simulink model "es2_emg_1"  (R2024a)
settings: Solver=VariableStepAuto  StartTime=0.0  StopTime=30  RelTol=1e-3
libraries: vrlib x2
settings Model: Creator=amisq  LastModifiedBy=amisq

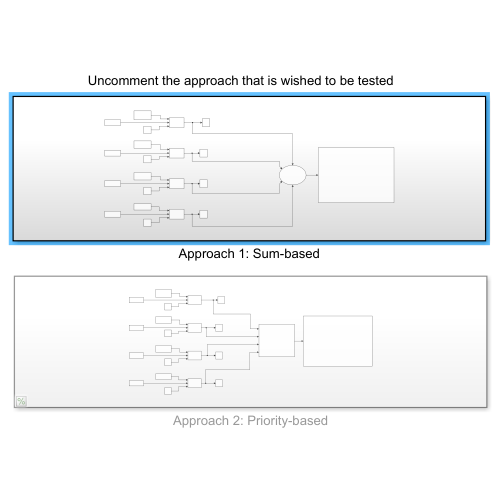
[thumbnail: Simulink's stored preview of the top-level diagram]
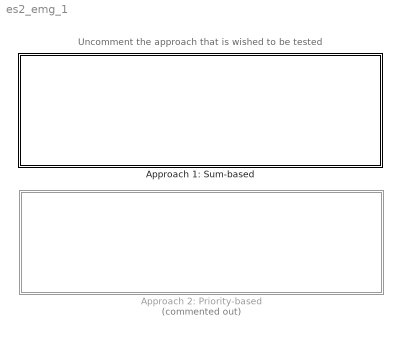
== system es2_emg_1 ==
  note: Uncomment the approach that is wished to be tested
  Approach 1: Sum-based : Subsystem
  Approach 2: Priority-based : Subsystem  Commented=on

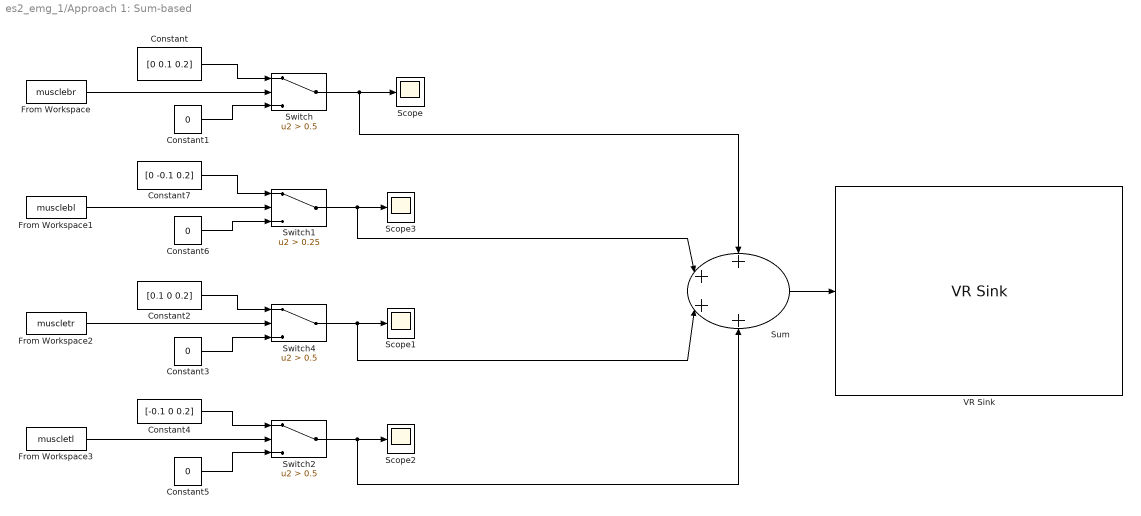
== system es2_emg_1/Approach 1: Sum-based ==
  Constant : Constant  Value=[0 0.1 0.2]
  Constant{1,3,5..6} (4 alike) : Constant  Value=0
  Constant2 : Constant  Value=[0.1 0 0.2]
  Constant4 : Constant  Value=[-0.1 0 0.2]
  Constant7 : Constant  Value=[0 -0.1 0.2]
  From Workspace : FromWorkspace  VariableName=musclebr  SampleTime=0.05
  From Workspace1 : FromWorkspace  VariableName=musclebl  SampleTime=0.05
  From Workspace2 : FromWorkspace  VariableName=muscletr  SampleTime=0.05
  From Workspace3 : FromWorkspace  VariableName=muscletl  SampleTime=0.05
  Scope{,1..3} (4 alike) : Scope
  Sum : Sum  Inputs=++++
  Switch : Switch  Criteria=u2 > Threshold  Threshold=0.5  SaturateOnIntegerOverflow=off  InputSameDT=off
  Switch1 : Switch  Criteria=u2 > Threshold  Threshold=0.25  SaturateOnIntegerOverflow=off  InputSameDT=off
  Switch2 : Switch  Criteria=u2 > Threshold  Threshold=0.5  SaturateOnIntegerOverflow=off  InputSameDT=off
  Switch4 : Switch  Criteria=u2 > Threshold  Threshold=0.5  SaturateOnIntegerOverflow=off  InputSameDT=off
  VR Sink : vrlib/VR Sink  InstantiateOnLoad=on  SampleTime=0.03  ViewEnable=on  RemoteChange=off  RemoteView=off  FieldsWritten=cursor.translation.3.1.1.double  WorldFileName=8_palline_color.wrl  AutoView=off  VideoDimensions=[]  AllowVariableSize=off
  wires:
  Switch2/1 -> Sum/4, Scope2/1
  Constant/1 -> Switch/1
  Switch/1 -> Sum/1, Scope/1
  From Workspace3/1 -> Switch2/2
  Constant2/1 -> Switch4/1
  Switch1/1 -> Sum/2, Scope3/1
  Constant4/1 -> Switch2/1
  Constant6/1 -> Switch1/3
  From Workspace1/1 -> Switch1/2
  Constant5/1 -> Switch2/3
  Constant7/1 -> Switch1/1
  Constant3/1 -> Switch4/3
  From Workspace2/1 -> Switch4/2
  Switch4/1 -> Sum/3, Scope1/1
  From Workspace/1 -> Switch/2
  Sum/1 -> VR Sink/1
  Constant1/1 -> Switch/3

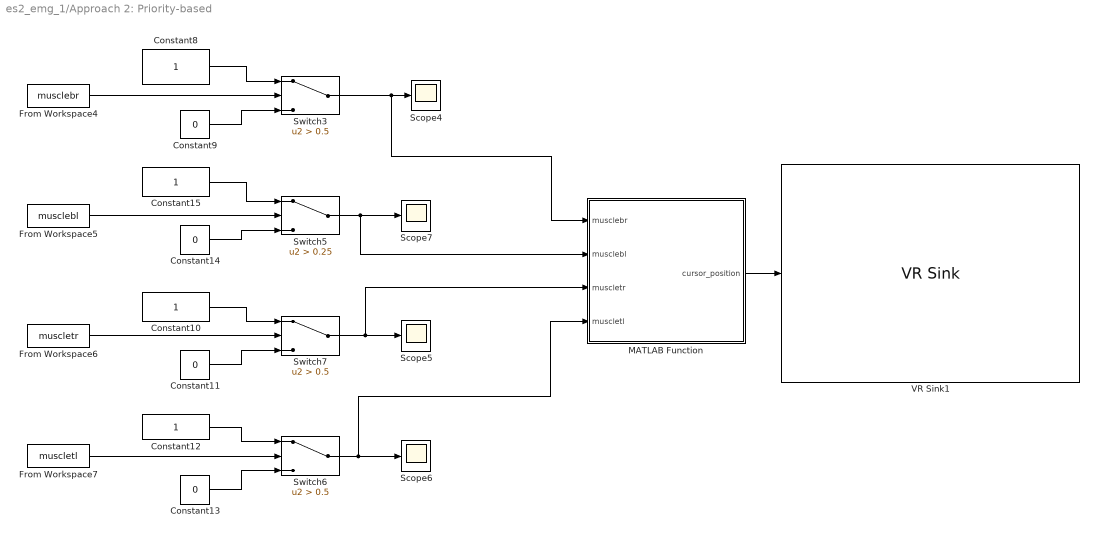
== system es2_emg_1/Approach 2: Priority-based ==
  Constant{8,10,12,15} (4 alike) : Constant
  Constant{9,11,13..14} (4 alike) : Constant  Value=0
  From Workspace4 : FromWorkspace  VariableName=musclebr  SampleTime=0.05
  From Workspace5 : FromWorkspace  VariableName=musclebl  SampleTime=0.05
  From Workspace6 : FromWorkspace  VariableName=muscletr  SampleTime=0.05
  From Workspace7 : FromWorkspace  VariableName=muscletl  SampleTime=0.05
  MATLAB Function : MATLAB Function  TreatAsAtomicUnit=on
  Scope{4..7} (4 alike) : Scope
  Switch3 : Switch  Criteria=u2 > Threshold  Threshold=0.5  SaturateOnIntegerOverflow=off  InputSameDT=off
  Switch5 : Switch  Criteria=u2 > Threshold  Threshold=0.25  SaturateOnIntegerOverflow=off  InputSameDT=off
  Switch6 : Switch  Criteria=u2 > Threshold  Threshold=0.5  SaturateOnIntegerOverflow=off  InputSameDT=off
  Switch7 : Switch  Criteria=u2 > Threshold  Threshold=0.5  SaturateOnIntegerOverflow=off  InputSameDT=off
  VR Sink1 : vrlib/VR Sink  InstantiateOnLoad=on  SampleTime=0.03  ViewEnable=on  RemoteChange=off  RemoteView=off  FieldsWritten=cursor.translation.3.1.1.double  WorldFileName=8_palline_color.wrl  AutoView=off  VideoDimensions=[]  AllowVariableSize=off
  wires:
  From Workspace4/1 -> Switch3/2
  From Workspace7/1 -> Switch6/2
  Switch6/1 -> MATLAB Function/4(muscletl), Scope6/1
  Constant11/1 -> Switch7/3
  MATLAB Function/1(cursor_position) -> VR Sink1/1
  Constant14/1 -> Switch5/3
  Constant15/1 -> Switch5/1
  Switch5/1 -> MATLAB Function/2(musclebl), Scope7/1
  Switch3/1 -> MATLAB Function/1(musclebr), Scope4/1
  Constant9/1 -> Switch3/3
  Constant12/1 -> Switch6/1
  Constant8/1 -> Switch3/1
  From Workspace5/1 -> Switch5/2
  Constant13/1 -> Switch6/3
  Switch7/1 -> Scope5/1, MATLAB Function/3(muscletr)
  From Workspace6/1 -> Switch7/2
  Constant10/1 -> Switch7/1

== matlab function es2_emg_1/Approach 2: Priority-based/MATLAB Function ==
  data: musclebr input; cursor_position output; musclebl input; muscletr input; muscletl input
function cursor_position = control_cursor(musclebr, musclebl, muscletr, muscletl)
    % Define the position vectors for the cardinal directions
    up = [0, 0.1, 0.2];     % Muscle 1 (up)
    down = [0, -0.1, 0.2];  % Muscle 2 (down)
    right = [0.1, 0, 0.2];  % Muscle 3 (right)
    left = [-0.1, 0, 0.2];  % Muscle 4 (left)

    % Priority system: prioritize muscles in a specific order
    if musclebl
        cursor_position = down; % Priority 1: Down
    elseif musclebr
        cursor_position = up; % Priority 2: Up 
    elseif muscletr
        cursor_position = right; % Priority 3: Right
    elseif muscletl
        cursor_position = left; % Priority 4: Left
    else
        cursor_position = [0, 0, 0.2]; % No muscles active, no movement
    end
end
